simulink model "Ej4_CruiseCtrl_StateFeedback"  (Simulink 9.1)
settings: Solver=ode45  StartTime=0.0  StopTime=100  MaxStep=0.01  RelTol=1e-3  EnableMultiTasking=on
values from neighbouring files (symbols this model uses):
  A = [ -ds/(Jf*i^2) ds/(Jf*i) -cs/(Jf*i) ... (first row only)    [Ej2.m]    (also in Ej4.m = [ -1.25       0)
  alpha = 0    [Ej4.m]
  B_d = [0 -1/Jc 0]'    [Ej2.m]    (also in Ej4.m = [0 -9.82]')
  B_u = [20000 0]'    [Ej4.m]
  C_ss = eye(2)    [Ej4.m]
  K = acker(A, B, P)    [Ej2.m]    (also in Ej4.m = acker(A, B_u, P))
  kr = -inv((C/(A-B*K))*B)    [Ej2.m]    (also in Ej4.m = -1/((C/(A-B_u*K))*B_u))
  ref_at1 = 20    [Ej4.m]
  ue = 0    [Ej4.m]
  x1e = 0    [Ej4.m]
  x2e = 0    [Ej4.m]
settings Model: Creator=JonasMac  LastModifiedBy=joses
settings DataIOCC: LimitDataPoints=on
settings DebuggingCC: SolverPrmCheckMsg=warning
settings GRTTargetCC: CombineOutputUpdateFcns=on  GRTInterface=off

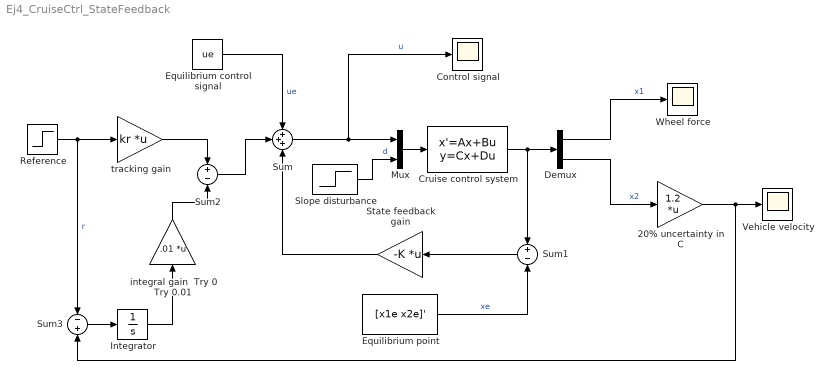
== system Ej4_CruiseCtrl_StateFeedback ==
  20% uncertainty in C : Gain  Gain=1.2  Multiplication=Matrix(K*u)
  Control signal : Scope
  Cruise control system : StateSpace  A=A  B=[B_u B_d]  C=C_ss  D=zeros(2)
  Demux : Demux  Outputs=2
  Equilibrium control signal : Constant  Value=ue
  "Equilibrium point " : Constant  Value=[x1e x2e]'
  Integrator : Integrator
  Mux : Mux  Inputs=2
  Reference : Step  Time=0  After=ref_at1  SampleTime=0
  Slope disturbance : Step  Time=20  After=sin(alpha)  SampleTime=0
  State feedback gain : Gain  Gain=-K  Multiplication=Matrix(K*u)
  Sum : Sum  Inputs=+++
  Sum1 : Sum  Inputs=+-
  Sum2 : Sum  Inputs=+-
  Sum3 : Sum  Inputs=-+
  Vehicle velocity : Scope
  Wheel force : Scope
  integral gain  Try 0 Try 0.01 : Gain  Gain=.01  Multiplication=Matrix(K*u)
  tracking gain : Gain  Gain=kr  Multiplication=Matrix(K*u)
  wires:
  Demux/1 -> Wheel force/1  "x1"
  Demux/2 -> 20% uncertainty in C/1  "x2"
  Sum/1 -> Mux/1, Control signal/1  "u"
  Slope disturbance/1 -> Mux/2  "d"
  Equilibrium control signal/1 -> Sum/1  "ue"
  Cruise control system/1 -> Sum1/1, Demux/1
  Mux/1 -> Cruise control system/1
  State feedback gain/1 -> Sum/3
  Sum1/1 -> State feedback gain/1
  "Equilibrium point "/1 -> Sum1/2  "xe"
  Reference/1 -> tracking gain/1, Sum3/1  "r"
  tracking gain/1 -> Sum2/1
  Sum2/1 -> Sum/2
  integral gain  Try 0 Try 0.01/1 -> Sum2/2
  Sum3/1 -> Integrator/1
  20% uncertainty in C/1 -> Sum3/2, Vehicle velocity/1
  Integrator/1 -> integral gain  Try 0 Try 0.01/1
